simulink subsystem "Day2_Scenario_4_5"  (R2024a)
settings: Solver=VariableStepAuto  StartTime=0.0  StopTime=10.0  RelTol=1e-3
undefined symbols (not defined in the file or in its folder): route1_waypoint_raw
libraries: CarMaker4SL x6, slpidlib x1
settings Model: Creator=junhyung.cha  LastModifiedBy=User

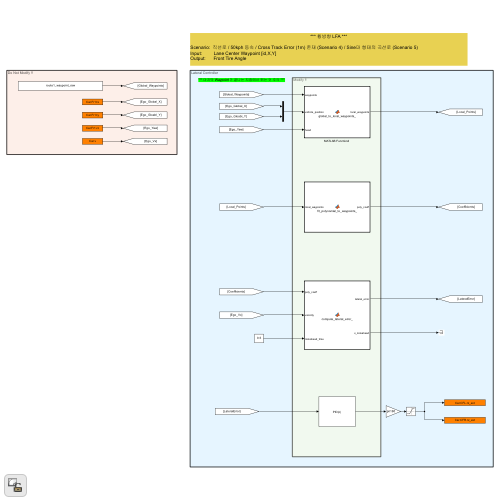
[thumbnail: Simulink's stored preview of the top-level diagram]
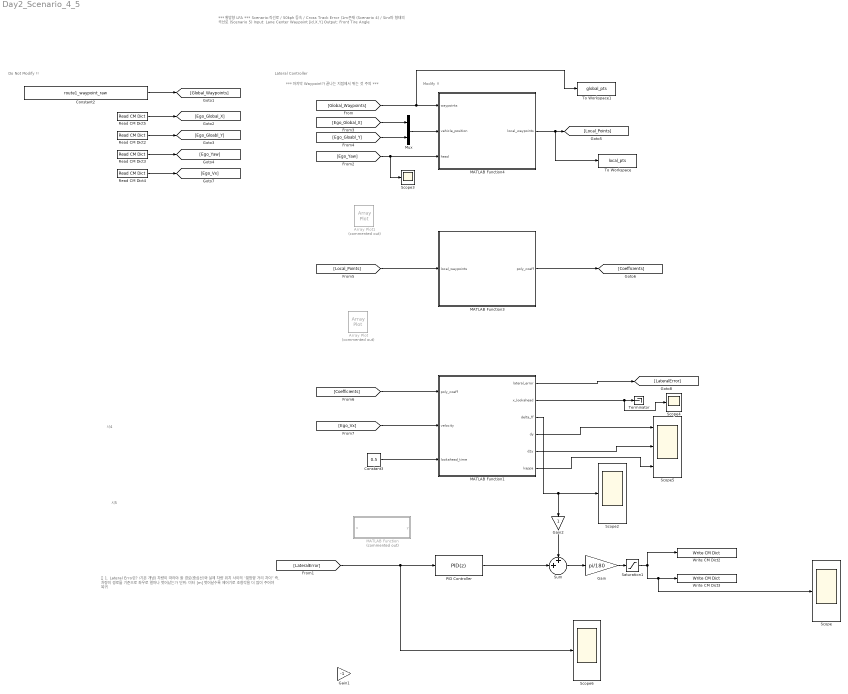
== system Day2_Scenario_4_5 ==
  note: 시4
  note: ✅ 1. Lateral Error란? (기본 개념)
      | 차량이 따라야 할 경로(중심선)와 실제 차량 위치 사이의 “횡방향 거리 차이”
      | 즉,
      | 차량이 경로를 기준으로 좌우로 얼마나 벗어났는가
      | 단위: 미터 [m]
      | 벗어날수록 제어기로 조향각을 더 많이 주어야 복귀
  note: *** 마지막 Waypoint가 끝나는 지점에서 튀는 것 주의 ***
  note: Modify !!
  note: Lateral Controller
  note: Do Not Modify !!
  note: *** 횡방향 LFA ***
      |
      | Scenario: 직선로 / 50kph 등속 / Cross Track Error (1m) 존재 (Scenario 4) / Sine파 형태의 곡선로 (Scenario 5)
      | Input: Lane Center Waypoint [id,X,Y]
      | Output: Front Tire Angle
  note: 시5
  Array Plot : ArrayPlot  Commented=on  ScopeFrameLocation=window  YLimits=[-550.9276 67.2813]  ShowLegend=on  ExpandToolstrip=on
  Array Plot1 : ArrayPlot  Commented=on  ScopeFrameLocation=window  YLimits=[-550.9276 67.2813]  ShowLegend=on  ExpandToolstrip=on
  Constant2 : Constant  Value=route1_waypoint_raw
  Constant3 : Constant  Value=0.5
  Gain : Gain  Gain=pi/180
  Gain1 : Gain  Gain=-1
  Gain2 : Gain
  MATLAB Function : MATLAB Function  Commented=on  TreatAsAtomicUnit=on
  MATLAB Function1 : MATLAB Function  TreatAsAtomicUnit=on
  MATLAB Function3 : MATLAB Function  TreatAsAtomicUnit=on
  "MATLAB Function4 " : MATLAB Function  TreatAsAtomicUnit=on
  Mux : Mux  Inputs=2
  PID Controller : slpidlib/PID Controller  Controller=PID  Form=Ideal  TimeDomain=Discrete-time  UseExternalTs=off  SampleTime=-1  IntegratorMethod=Forward Euler  FilterMethod=Forward Euler  ControllerParametersSource=internal  P=3  I=2  UseKiTs=off  D=1.5  UseExternalDerivativeSource=off  N=1000  UseFilter=off  TunerSelectOption=Transfer Function Based (PID Tuner App)  InitialConditionSource=internal  InitialConditionForIntegrator=0  InitialConditionForFilter=0  DifferentiatorICPrevScaledInput=0  ExternalReset=none  TrackingMode=off  Kt=1  LimitOutput=off  SatLimitsSource=internal  UpperSaturationLimit=1  LowerSaturationLimit=-1  LinearizeAsGain=on  AntiWindupMode=back-calculation  Kb=1  LimitIntegrator=off  UpperIntegratorSaturationLimit=0.7  LowerIntegratorSaturationLimit=-0.7  POutMin=[]  POutMax=[]  IOutMin=[]  IOutMax=[]  DOutMin=[]  DOutMax=[]  NOutMin=[]  NOutMax=[]  SumOutMin=[]  SumOutMax=[]  SaturationOutMin=[]  SaturationOutMax=[]  PParamMin=[]  PParamMax=[]  IParamMin=[]  IParamMax=[]  DParamMin=[]  DParamMax=[]  NParamMin=[]  NParamMax=[]  KbParamMin=[]  KbParamMax=[]  KtParamMin=[]  KtParamMax=[]  KbOutMin=[]  KbOutMax=[]  KtOutMin=[]  KtOutMax=[]  IntegratorOutMin=[]  IntegratorOutMax=[]  FilterOutMin=[]  FilterOutMax=[]  SumI1OutMin=[]  SumI1OutMax=[]  SumI2OutMin=[]  SumI2OutMax=[]  SumI3OutMin=[]  SumI3OutMax=[]  SumI4OutMin=[]  SumI4OutMax=[]  SumDOutMin=[]  SumDOutMax=[]  DifferentiatorOutMin=[]  DifferentiatorOutMax=[]  FilterDiffOutCoefMin=[]  FilterDiffOutCoefMax=[]  ReciprocalOutMin=[]  ReciprocalOutMax=[]  SumDenOutMin=[]  SumDenOutMax=[]  SumNumOutMin=[]  SumNumOutMax=[]  DivideOutMin=[]  DivideOutMax=[]  UdiffTsProdOutMin=[]  UdiffTsProdOutMax=[]  NTsProdOutMin=[]  NTsProdOutMax=[]  UintegralTsProdOutMin=[]  UintegralTsProdOutMax=[]  UngainTsProdOutMin=[]  UngainTsProdOutMax=[]  ClampingZeroOutDataTypeStr=Inherit: Inherit via back propagation  ClampingZeroOutMin=[]  ClampingZeroOutMax=[]  FilterDenConstantOutDataTypeStr=Inherit: Inherit via back propagation  FilterDenConstantOutMin=[]  FilterDenConstantOutMax=[]  PCopyOutDataTypeStr=Inherit: Inherit via back propagation  PCopyOutMin=[]  PCopyOutMax=[]  NCopyOutDataTypeStr=Inherit: Inherit via back propagation  NCopyOutMin=[]  NCopyOutMax=[]  IntegratorContinuousStateAttributes=''  IntegratorStateMustResolveToSignalObject=off  IntegratorRTWStateStorageClass=Auto  FilterContinuousStateAttributes=''  FilterStateMustResolveToSignalObject=off  FilterRTWStateStorageClass=Auto  ParallelPVariant=Passthrough  IdealPVariant=InternalParameters  IVariant=InternalParameters  DVariant=InternalParameters  IntegratorVariant=Discrete  SatVariant=Disabled  AWVariant=Passthrough  PCopyVariant=Disabled  TRVariant=Disabled  FdbkBlocksVariant=Forward  IdealPFdbkVariant=Disabled  SatFdbkVariant=Disabled  DerivativeFilterVariant=Differentiator  NVariant=Passthrough  NCopyVariant=Disabled_SignalSpec  FilterICVariant=InternalICsDifferentiator  IntegratorICVariant=InternalICs  ExternalResetVariant=Disabled  TRSumVariant=Passthrough  SumFdbkVariant=Disabled  SumVariant=Sum_PID  TsampFilterVariant=InternalTs  TsampNgainVariant=Passthrough  TsampIntegralVariant=Disabled_SignalSpec  ExternalSaturationOutDataTypeStr=Inherit: Same as second input  DerivativeSourceVariant=ErrorSignal
  Read CM Dict2 : CarMaker4SL/Read CM Dict  xname=Car.Fr1.ty  xsync=off  xstime=Inherited
  Read CM Dict3 : CarMaker4SL/Read CM Dict  xname=Car.Fr1.rz  xsync=off  xstime=Inherited
  Read CM Dict4 : CarMaker4SL/Read CM Dict  xname=Car.v  xsync=off  xstime=Inherited
  Read CM Dict5 : CarMaker4SL/Read CM Dict  xname=Car.Fr1.tx  xsync=off  xstime=Inherited
  Saturation1 : Saturate
  Scope{,2..4,6} (5 alike) : Scope
  Scope5 : Scope  NumInputPorts=3
  Sum : Sum  Inputs=++|
  Terminator : Terminator
  To Workspace : ToWorkspace  VariableName=local_pts  SampleTime=-1
  To Workspace1 : ToWorkspace  VariableName=global_pts  SampleTime=-1
  Write CM Dict2 : CarMaker4SL/Write CM Dict  xname=Car.CFL.rz_ext  xsync=off
  Write CM Dict3 : CarMaker4SL/Write CM Dict  xname=Car.CFR.rz_ext  xsync=off
  wires:
  Read CM Dict5/1 -> [Ego_Global_X]
  Read CM Dict2/1 -> [Ego_Gloabl_Y]
  Read CM Dict3/1 -> [Ego_Yaw]
  [Ego_Yaw] -> "MATLAB Function4 "/3(head), Scope3/1
  [Ego_Global_X] -> Mux/1
  [Ego_Gloabl_Y] -> Mux/2
  "MATLAB Function4 "/1(local_waypoints) -> [Local_Points], To Workspace/1
  [Local_Points] -> MATLAB Function3/1(local_waypoints)
  MATLAB Function3/1(poly_coeff) -> [Coefficients]
  [Coefficients] -> MATLAB Function1/1(poly_coeff)
  Constant3/1 -> MATLAB Function1/3(lookahead_time)
  Saturation1/1 -> Write CM Dict3/1, Scope/1, Write CM Dict2/1
  MATLAB Function1/1(lateral_error) -> [LateralError]
  [Ego_Vx] -> MATLAB Function1/2(velocity)
  Mux/1 -> "MATLAB Function4 "/2(vehicle_position)
  Read CM Dict4/1 -> [Ego_Vx]
  MATLAB Function1/2(x_lookahead) -> Terminator/1, Scope4/1
  [Global_Waypoints] -> "MATLAB Function4 "/1(waypoints), To Workspace1/1
  Sum/1 -> Gain/1
  MATLAB Function1/3(delta_ff) -> Scope2/1, Gain2/1
  MATLAB Function1/4(dy) -> Scope5/1
  MATLAB Function1/5(d2y) -> Scope5/2
  MATLAB Function1/6(kappa) -> Scope5/3
  Constant2/1 -> [Global_Waypoints]
  [LateralError] -> Scope6/1, PID Controller/1
  PID Controller/1 -> Sum/2
  Gain/1 -> Saturation1/1
  Gain2/1 -> Sum/1

== matlab function Day2_Scenario_4_5/MATLAB Function ==
  data: u input; y output
function y = fcn(u)
% u: Lateral Error
% y: 조향각 제어 출력 (deg 단위, 최종적으로 rad 변환됨)

% 파라미터 설정 (게인 값은 시뮬레이션 보고 튜닝)
Kp = 0.3;     % 비례 이득
Kd = 0.0001;     % 미분 이득

% 상태 유지용 persistent 변수
persistent prev_error dt
if isempty(prev_error)
    prev_error = 0;
end
if isempty(dt)
    dt = 0.001;  % 샘플링 시간 (초)
end

% 오차 변화율 계산
derivative = (u - prev_error) / dt;

% PD 제어 계산
y = Kp * u + Kd * derivative;

% 이전 오차 업데이트
prev_error = u;
end

== matlab function Day2_Scenario_4_5/MATLAB Function1 ==
  settings: updateMethod=DISCRETE
  data: poly_coeff input; lateral_error output; velocity input; lookahead_time input; x_lookahead output; delta_ff output; dy output; d2y output; kappa output
% function [lateral_error, x_lookahead] = compute_lateral_error_(poly_coeff, velocity, lookahead_time)
% % ------------------------------------------------------------
% % 차량의 Lookahead 위치에서의 횡방향 오차 계산
% % 입력:
% %   - poly_coeff: 2차 다항식 계수 [a b c] (y = ax^2 + bx + c)
% %   - velocity: 차량 속도 [m/s]
% %   - lookahead_time: 전방 예측 시간 [s]
% % 출력:
% %   - lateral_error: lookahead 지점에서 차선 중심으로부터의 y 오차
% %   - x_lookahead: 차량 전방 예측 거리 (= velocity * lookahead_time)
% % ------------------------------------------------------------
% 
% % 예측 거리 = 현재 속도 × 예측 시간
% x_lookahead = velocity * lookahead_time;
% 
% % 예측 지점에서의 차선 중심 좌표 (y = ax^2 + bx + c)
% lateral_error = polyval(poly_coeff, x_lookahead);
% 
% end


% function [lateral_error, x_lookahead] = compute_lateral_error_(poly_coeff, velocity, lookahead_time)
% 
% % Lookahead 거리 계산
% x = velocity * lookahead_time;
% 
% % 다항식 계수
% a2 = poly_coeff(1);
% a1 = poly_coeff(2);
% a0 = poly_coeff(3);
% 
% % 경로 상 y 값 계산
% y = polyval(poly_coeff, x);  % 경로 위 y 좌표
% 
% % 도함수, 이차 도함수
% dy = 2 * a2 * x + a1;
% d2y = 2 * a2;
% 
% % 곡률 계산
% kappa = d2y / (1 + dy^2)^(3/2);
% 
% % lateral error = 경로 y 좌표 - 차량 위치(y=0)
% lateral_error = y;
% 
% % x_lookahead에 x와 곡률을 담아서 전달
% x_lookahead = [x, kappa];
% 
% end
%% 


% % function [lateral_error, x_lookahead, delta_ff] = compute_lateral_error_(poly_coeff, velocity, lookahead_time)
% function [lateral_error, x_lookahead, delta_ff, dy, d2y, kappa] = compute_lateral_error_(poly_coeff, velocity, lookahead_time)
% % Lookahead x 계산
% x_lookahead = velocity * lookahead_time;
% 
% % 계수 초기화
% a = 0; b = 0; c = 0; d = 0;
% n = length(poly_coeff);
% 
% if n == 4         % 3차 다항식
%     a = poly_coeff(1);
%     b = poly_coeff(2);
%     c = poly_coeff(3);
%     d = poly_coeff(4);
% elseif n == 3     % 2차
%     b = poly_coeff(1);
%     c = poly_coeff(2);
%     d = poly_coeff(3);
% elseif n == 2     % 1차
%     c = poly_coeff(1);
%     d = poly_coeff(2);
% elseif n == 1     % 상수
%     d = poly_coeff(1);
% end
% 
% % 예측 위치에서의 y값 → lateral error
% y_lookahead = a*x_lookahead^3 + b*x_lookahead^2 + c*x_lookahead + d;
% lateral_error = y_lookahead;   % ego 차량은 항상 y = 0
% 
% % Feedforward 조향각 계산 (정확한 곡률 기반)
% dy  = 3*a*x_lookahead^2 + 2*b*x_lookahead + c;   % 1차 미분 (y')
% d2y = 6*a*x_lookahead + 2*b;                     % 2차 미분 (y'')
% 
% kappa = d2y / (1 + dy^2)^(3/2);  % 곡률 공식
% L = 2.9;                         % wheelbase [m]
% delta_ff = atan(L * kappa);     % 조향각
% 
% end

%% 
% function [lateral_error, x_lookahead, delta_ff, dy, d2y, kappa] = compute_lateral_error_(poly_coeff, velocity, lookahead_time)
% 
% % Lookahead x 계산
% x_lookahead = velocity * lookahead_time;
% 
% % 계수 길이 확인
% n = length(poly_coeff);
% a = 0; b = 0; c = 0;
% if n == 4
%     a = poly_coeff(1);
%     b = poly_coeff(2);
%     c = poly_coeff(3);
%     d = poly_coeff(4);
% elseif n == 3
%     b = poly_coeff(1); c = poly_coeff(2); d = poly_coeff(3);
% elseif n == 2
%     c = poly_coeff(1); d = poly_coeff(2);
% else
%     d = poly_coeff(1);
% end
% 
% % y(x) 계산 → lateral error
% lateral_error = a*x_lookahead^3 + b*x_lookahead^2 + c*x_lookahead + d;
% 
% % 1차, 2차 도함수
% dy = 3*a*x_lookahead^2 + 2*b*x_lookahead + c;
% d2y = 6*a*x_lookahead + 2*b;
% 
% % 곡률 계산
% denominator = (1 + dy^2)^(3/2);
% if denominator < 1e-6
%     denominator = 1e-6;  % 0으로 나누기 방지
% end
% kappa = d2y / denominator;
% 
% % Feedforward
% L = 2.9;
% delta_ff = atan(L * kappa);
% 
% end


%% 
% function [lateral_error, x_lookahead, delta_ff, dy, d2y, kappa] = compute_lateral_error_(poly_coeff, velocity, lookahead_time)
% % ------------------------------------------------------------
% % 경로 다항식 기반 곡률 및 조향각 계산
% % ------------------------------------------------------------
% % 입력:
% %   - poly_coeff: 다항식 계수 [a b c d]
% %   - velocity: 현재 속도 (m/s)
% %   - lookahead_time: 미리 볼 시간 (s)
% %
% % 출력:
% %   - lateral_error: y(0) → 현 위치에서 횡방향 오차
% %   - x_lookahead: vx * lookahead_time
% %   - delta_ff: Feedforward 조향각 (rad)
% %   - dy, d2y: 1차, 2차 미분값
% %   - kappa: 곡률
% % ------------------------------------------------------------
% 
% % 차량 휠베이스 (L) [필요시 수정]
% L = 3;  % 단위: meter
% 
% % 다항식 계수 추출
% a = poly_coeff(1);
% b = poly_coeff(2);
% c = poly_coeff(3);
% d = poly_coeff(4);
% 
% % 1. 현재 위치 횡방향 오차
% lateral_error = d;  % 차량 기준 위치는 x=0이므로 y(0) = d
% 
% % 2. lookahead 위치 계산
% x_lookahead = velocity * lookahead_time;
% 
% % 3. 1차 및 2차 미분값 (예측 지점에서)
% dy = 3*a*x_lookahead^2 + 2*b*x_lookahead + c;
% d2y = 6*a*x_lookahead + 2*b;
% 
% % 4. 곡률 계산
% kappa = d2y / (1 + dy^2)^(3/2);
% 
% % 5. 조향각 계산 (작은 각도 근사 또는 atan 사용 가능)
% delta_ff = L * kappa;  % 또는 atan(L * kappa)
% 
% end



%% 
% function [lateral_error, x_lookahead, delta_ff, dy, d2y, kappa] = compute_lateral_error_(poly_coeff, velocity, lookahead_time)
% % ------------------------------------------------------------
% % 경로 다항식 기반 곡률 및 조향각 계산
% % ------------------------------------------------------------
% % 입력:
% %   - poly_coeff: 다항식 계수 [a b c d] (3차 다항식)
% %   - velocity: 현재 속도 (m/s)
% %   - lookahead_time: 미리 볼 시간 (s)
% %
% % 출력:
% %   - lateral_error: y(0) → 현 위치에서 횡방향 오차
% %   - x_lookahead: vx * lookahead_time
% %   - delta_ff: Feedforward 조향각 (rad)
% %   - dy, d2y: 1차, 2차 미분값
% %   - kappa: 곡률
% % ------------------------------------------------------------
% 
% % 차량 휠베이스 (m)
% L = 3.0;
% 
% % 다항식 계수 추출 (차수 부족 대비)
% a = 0; b = 0; c = 0; d = 0;
% n = length(poly_coeff);
% 
% if n == 4
%     a = poly_coeff(1); b = poly_coeff(2); c = poly_coeff(3); d = poly_coeff(4);
% elseif n == 3
%     b = poly_coeff(1); c = poly_coeff(2); d = poly_coeff(3);
% elseif n == 2
%     c = poly_coeff(1); d = poly_coeff(2);
% elseif n == 1
%     d = poly_coeff(1);
% end
% 
% % 1. 현재 위치 횡방향 오차 (x = 0 → y = d)
% lateral_error = d;
% 
% % 2. 예측 거리 계산
% x_lookahead = velocity * lookahead_time;
% 
% % 3. 1차 및 2차 미분 계산
% dy = 3*a*x_lookahead^2 + 2*b*x_lookahead + c;
% d2y = 6*a*x_lookahead + 2*b;
% 
% % 4. 곡률 계산: 수치 안정성 확보
% denominator = (1 + dy^2)^(3/2);
% if denominator < 1e-6
%     denominator = 1e-6;  % 0 나누기 방지
% end
% kappa = d2y / denominator;
% 
% % 5. Feedforward 조향각 계산 (작은 각도 근사 또는 atan 사용)
% delta_ff = L * kappa;         % 단위: rad (작은 각도 근사)
% % delta_ff = atan(L * kappa); % <- 더 정확한 계산 (필요시 교체)
% 
% end
% 



%% 
% 
% function [lateral_error, x_lookahead, delta_ff, dy, d2y, kappa] = compute_lateral_error_(poly_coeff, velocity, lookahead_time)
% % ------------------------------------------------------------
% % 경로 다항식 기반 곡률 및 조향각 계산 (스무딩 포함)
% % ------------------------------------------------------------
% 
% % 휠베이스
% L = 3.0;
% 
% % 다항식 계수 추출
% a = 0; b = 0; c = 0; d = 0;
% n = length(poly_coeff);
% if n == 4
%     a = poly_coeff(1); b = poly_coeff(2); c = poly_coeff(3); d = poly_coeff(4);
% elseif n == 3
%     b = poly_coeff(1); c = poly_coeff(2); d = poly_coeff(3);
% elseif n == 2
%     c = poly_coeff(1); d = poly_coeff(2);
% else
%     d = poly_coeff(1);
% end
% 
% % 1. lateral error (x = 0)
% lateral_error = d;
% 
% % 2. lookahead 위치
% x_lookahead = velocity * lookahead_time;
% 
% % 3. dy, d2y
% dy = 3*a*x_lookahead^2 + 2*b*x_lookahead + c;
% d2y = 6*a*x_lookahead + 2*b;
% 
% % 4. kappa 계산
% denominator = (1 + dy^2)^(3/2);
% if denominator < 1e-6
%     denominator = 1e-6;
% end
% kappa = d2y / denominator;
% 
% % 5. delta_ff 계산 (rad 기준)
% delta_now = L * kappa;
% 
% % 6. Moving Average Filter 적용
% persistent delta_buffer
% if isempty(delta_buffer)
%     delta_buffer = zeros(1, 30);  % 최근 5개 저장
% end
% 
% % shift + 최신값 추가
% delta_buffer = [delta_now, delta_buffer(1:end-1)];
% 
% % 평균값 출력
% delta_ff = mean(delta_buffer);
% 
% end
% 


%% 
function [lateral_error, x_lookahead, delta_ff, dy, d2y, kappa] = compute_lateral_error_(poly_coeff, velocity, lookahead_time)
% ------------------------------------------------------------
% 경로 다항식 기반 곡률 및 조향각 계산 (스무딩 포함)
% Waypoint 부족 시 조향각 0 처리
% ------------------------------------------------------------

% 휠베이스
L = 3.0;

% Waypoint 부족으로 poly_coeff가 모두 0일 경우 → 계산 중단
if all(poly_coeff == 0)
    lateral_error = 0;
    x_lookahead = velocity * lookahead_time;
    delta_ff = 0;
    dy = 0;
    d2y = 0;
    kappa = 0;
    return;
end

% 다항식 계수 추출
a = 0; b = 0; c = 0; d = 0;
n = length(poly_coeff);
if n == 4
    a = poly_coeff(1); b = poly_coeff(2); c = poly_coeff(3); d = poly_coeff(4);
elseif n == 3
    b = poly_coeff(1); c = poly_coeff(2); d = poly_coeff(3);
elseif n == 2
    c = poly_coeff(1); d = poly_coeff(2);
else
    d = poly_coeff(1);
end

% 1. lateral error (x = 0)
lateral_error = d;

% 2. lookahead 위치
x_lookahead = velocity * lookahead_time;

% 3. dy, d2y
dy = 3*a*x_lookahead^2 + 2*b*x_lookahead + c;
d2y = 6*a*x_lookahead + 2*b;

% 4. kappa 계산 (수치 안정성 보장)
denominator = (1 + dy^2)^(3/2);
if denominator < 1e-6
    denominator = 1e-6;
end
kappa = d2y / denominator;

% 5. 조향각 계산
delta_now = L * kappa;

% 6. Moving Average Filter 적용 (스무딩)
persistent delta_buffer
if isempty(delta_buffer)
    delta_buffer = zeros(1, 30);  % 최근 30개 저장
end

% shift + 최신값 추가
delta_buffer = [delta_now, delta_buffer(1:end-1)];

% 평균값 출력
delta_ff = mean(delta_buffer);

end

== matlab function Day2_Scenario_4_5/MATLAB Function3 ==
  settings: updateMethod=DISCRETE
  data: local_waypoints input; poly_coeff output
% function poly_coeff  = fit_polynomial_to_waypoints_(local_waypoints)
% % ------------------------------------------------------------
% % 차량 기준 로컬 경로점을 3차 다항식으로 피팅 (Scenario 5 포함 대응)
% % ------------------------------------------------------------
% 
% x = local_waypoints(:,1);
% y = local_waypoints(:,2);
% 
% if length(x) >= 4
%     poly_coeff = polyfit(x, y, 3);  % [a b c d] → 3차 다항식
% else
%     poly_coeff = [0 0 0 0];  % fallback
% end
% end
%% 

% function poly_coeff = fit_polynomial_to_waypoints_(local_waypoints)
% % ------------------------------------------------------------
% % 차량 기준 로컬 경로점을 3차 다항식으로 피팅
% % x 거리 기준으로 일정 범위 내 포인트만 사용
% % ------------------------------------------------------------
% % 입력:
% %   - local_waypoints: [N x 2] (로컬 좌표계 상의 X, Y)
% % 출력:
% %   - poly_coeff: 다항식 계수 [a b c d] (3차 기준)
% % ------------------------------------------------------------
% 
% % 1. 피팅 대상 거리 설정 (앞쪽 20m 내 포인트만 사용)
% x_max = 20;  % 예: 20m 전방까지만 사용
% 
% % 2. 포인트 분리
% x_all = local_waypoints(:,1);
% y_all = local_waypoints(:,2);
% 
% % 3. 거리 기준 필터링: 0 < x < x_max 범위만
% idx = find(x_all > 0 & x_all < x_max);
% 
% x = x_all(idx);
% y = y_all(idx);
% 
% % 4. 충분한 포인트 수 확인 (최소 4개 이상 있어야 3차 가능)
% if length(x) >= 4
%     poly_coeff = polyfit(x, y, 3);  % [a b c d]
% else
%     poly_coeff = zeros(1, 4);  % 피팅 불가 시 0으로 대체
% end
% 
% end
% 

%% 
% function poly_coeff = fit_polynomial_to_waypoints_(local_waypoints)
% % ------------------------------------------------------------
% % 차량 기준 로컬 경로점을 3차 다항식으로 피팅
% % 거리 기반 필터링: 차량 전방 x=0~20m 구간만 사용
% % ------------------------------------------------------------
% % 입력:
% %   - local_waypoints: [N x 2] (로컬 좌표계 X, Y)
% % 출력:
% %   - poly_coeff: 다항식 계수 [a b c d] (3차 기준)
% % ------------------------------------------------------------
% 
% % 1. 사용할 거리 범위 설정 (예: 차량 전방 20m)
% x_min = 0;
% x_max = 20;
% 
% % 2. X, Y 분리
% x_all = local_waypoints(:, 1);
% y_all = local_waypoints(:, 2);
% 
% % 3. 거리 필터링: 전방 일정 범위 내 웨이포인트만 추출
% idx = find(x_all > x_min & x_all < x_max);
% 
% x = x_all(idx);
% y = y_all(idx);
% 
% % 4. 최소한의 점 수 확인 (3차 다항식에 최소 4개 필요)
% if length(x) >= 4
%     poly_coeff = polyfit(x, y, 3);  % 3차 다항식 → [a b c d]
% else
%     poly_coeff = zeros(1, 4);       % 불안정한 경우 0으로 대체
% end
% 
% end
% 


%% 

% function poly_coeff = fit_polynomial_to_waypoints(local_waypoints)
% % S자형 경로 대응용 다항식 피팅
% % 단, 앞쪽 일정 거리 (x > 0) 포인트만 사용
% 
% % 유효한 포인트 필터링 (정방향)
% valid_idx = local_waypoints(:,1) > 0;
% filtered = local_waypoints(valid_idx, :);
% 
% % 앞쪽 30개만 사용
% N = min(30, size(filtered, 1));
% x = filtered(1:N, 1);
% y = filtered(1:N, 2);
% 
% % 3차 다항식 피팅
% if length(x) >= 4
%     poly_coeff = polyfit(x, y, 3);
% else
%     poly_coeff = zeros(1,4);
% end
% end


%% 
% 
% function poly_coeff = fit_polynomial_to_waypoints(local_waypoints)
% %#codegen
% % fit_polynomial_to_waypoints - Sliding Window 기반 다항식 피팅
% %
% % 입력:
% %   local_waypoints : Nx2 matrix of [x, y] in vehicle-local frame
% % 출력:
% %   poly_coeff      : 1x4 vector [a3 a2 a1 a0] such that
% %                     y ≈ a3*x^3 + a2*x^2 + a1*x + a0
% 
%     %% 파라미터 (원하면 tunable parameter로 만들 수 있음)
%     max_distance = 15.0;   % 차량 전방 최대 거리 [m]
%     max_points   = 10;     % 최대 사용 포인트 수
%     poly_order   = 3;      % 다항식 차수 (3차)
% 
%     %% 1. x, y 분리
%     x_all = local_waypoints(:,1);
%     y_all = local_waypoints(:,2);
% 
%     %% 2. 전방 필터링: x > 0 이고 max_distance 이하
%     valid_idx = find(x_all > 0 & x_all < max_distance);
%     x_sel = x_all(valid_idx);
%     y_sel = y_all(valid_idx);
% 
%     %% 3. 최대 사용 포인트 제한
%     if length(x_sel) > max_points
%         x_sel = x_sel(1:max_points);
%         y_sel = y_sel(1:max_points);
%     end
% 
%     %% 4. 최소 포인트 조건 확인
%     if length(x_sel) < poly_order + 1
%         poly_coeff = zeros(1, poly_order + 1);  % 피팅 실패 시 0 반환
%         return;
%     end
% 
%     %% 5. 다항식 피팅
%     poly_coeff = polyfit(x_sel, y_sel, poly_order);
% end
% 


%% 

% function poly_coeff = fit_polynomial_to_waypoints_(local_waypoints)
% % ------------------------------------------------------------
% % 차량 기준 로컬 경로점을 3차 다항식으로 피팅
% % - X > 0 방향만 사용 (정방향)
% % - 최대 10개까지만 사용 (개수 기반)
% % - X < 15m 조건 추가 (거리 기반)
% % - 포인트 부족 시 안정적으로 0 반환
% % ------------------------------------------------------------
% % 입력:
% %   - local_waypoints: [N x 2] (로컬 좌표계 X, Y)
% % 출력:
% %   - poly_coeff: 다항식 계수 [a b c d] (3차 기준)
% % ------------------------------------------------------------
% 
% % 파라미터 설정
% poly_order = 3;        % 다항식 차수 (3차)
% max_points = 10;       % 사용할 최대 포인트 수
% x_limit = 15;          % 사용할 최대 X 거리
% 
% % 1. 정방향 웨이포인트만 필터링
% valid_idx = local_waypoints(:,1) > 0;
% filtered = local_waypoints(valid_idx, :);
% 
% % 2. 거리 제한 (x < x_limit)
% dist_idx = filtered(:,1) < x_limit;
% filtered = filtered(dist_idx, :);
% 
% % 3. 앞쪽 max_points개만 사용
% N = min(max_points, size(filtered, 1));
% x_sel = filtered(1:N, 1);
% y_sel = filtered(1:N, 2);
% 
% % 4. 최소 포인트 조건 확인
% if length(x_sel) < poly_order + 1
%     % Waypoint 부족 → 안전하게 y = 0 직선으로 가정
%     poly_coeff = [0 0 0 0];
%     return;
% end
% 
% % 5. 다항식 피팅
% poly_coeff = polyfit(x_sel, y_sel, poly_order);  % → [a b c d]
% 
% end


%% 
function poly_coeff = fit_polynomial_to_waypoints_(local_waypoints)

% 설정값
poly_order = 3;
max_points = 10;
x_limit = 20;
y_limit = 5;

% 1. x > 0, x < x_limit, |y| < y_limit 필터링
idx = find( ...
    local_waypoints(:,1) > 0 & ...
    local_waypoints(:,1) < x_limit & ...
    abs(local_waypoints(:,2)) < y_limit );

filtered = local_waypoints(idx, :);

% 2. 앞쪽 max_points개만 사용
N = min(max_points, size(filtered, 1));
x = filtered(1:N, 1);
y = filtered(1:N, 2);

% 3. 피팅 수행
if length(x) >= poly_order + 1
    poly_coeff = polyfit(x, y, poly_order);
else
    poly_coeff = zeros(1, 4);
end

end

== matlab function Day2_Scenario_4_5/MATLAB Function4  ==
  settings: updateMethod=DISCRETE
  data: waypoints input; local_waypoints output; vehicle_position input; head input

%% 

function local_waypoints = global_to_local_waypoints_(waypoints, vehicle_position, head)
% ------------------------------------------------------------
% Global waypoints → 차량 기준 local 좌표계 변환
% 끝부분 웨이포인트 제거 (예: 뒤에서 10개 제거)
% ------------------------------------------------------------

% 1. 끝부분 제거 (조건 없이 항상 10개 제거, 크기 고정되게)
waypoints = waypoints(1:end-50, :);

% 2. 차량 기준 좌표계 원점으로 이동
dx = waypoints(:,1) - vehicle_position(1);
dy = waypoints(:,2) - vehicle_position(2);

% 3. 회전 행렬 적용 (yaw만큼 반시계 회전)
local_x = dx .* cos(-head) - dy .* sin(-head);
local_y = dx .* sin(-head) + dy .* cos(-head);

% 4. 최종 로컬 웨이포인트 반환
local_waypoints = [local_x, local_y];

end
